simulink model "simu8"  (R2023b)
settings: Solver=VariableStepAuto  StartTime=0.0  StopTime=10.0  RelTol=1e-3
values from neighbouring files (symbols this model uses):
  b = 0.0012    [CFRO.m]    (also in parametros8.m)
  J = 0.001    [CFRO.m]    (also in parametros8.m)
  Ke = 0.01    [CFRO.m]    (also in parametros8.m)
  Kt = 0.01    [CFRO.m]    (also in parametros8.m)
  Lu = 0.023    [CFRO.m]    (also in parametros8.m)
  Ra = 2    [parametros8.m]

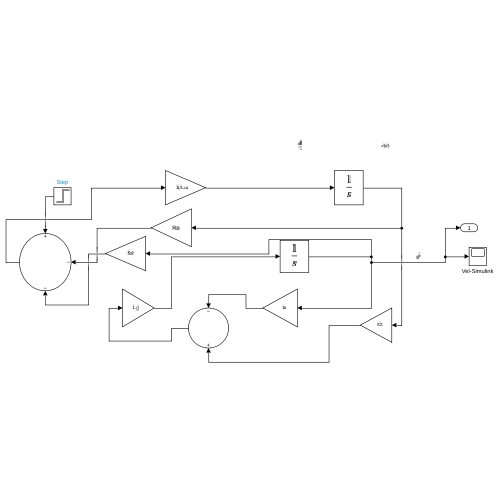
[thumbnail: Simulink's stored preview of the top-level diagram]
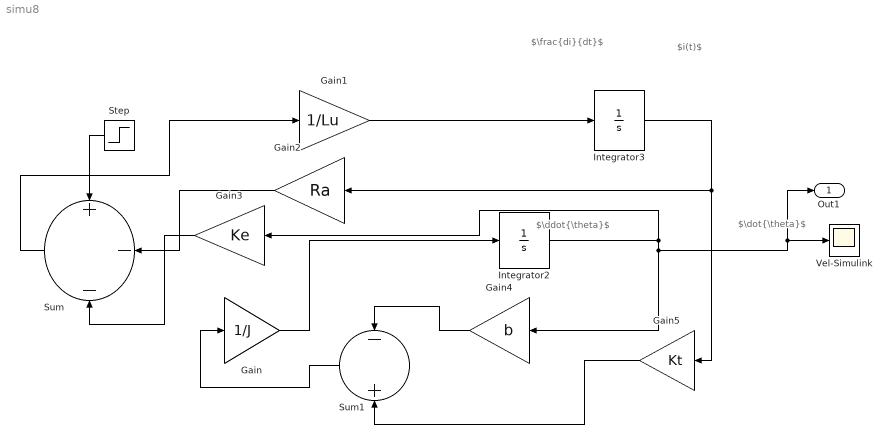
== system simu8 ==
  note: $\ddot{\theta}$
  note: $\frac{di}{dt}$
  note: $i(t)$
  note: $\dot{\theta}$
  Gain : Gain  Gain=1/J
  Gain1 : Gain  Gain=1/Lu
  Gain2 : Gain  Gain=Ra
  Gain3 : Gain  Gain=Ke
  Gain4 : Gain  Gain=b
  Gain5 : Gain  Gain=Kt
  Integrator2 : Integrator
  Integrator3 : Integrator
  Step : Step  Time=0  After=5  SampleTime=0
  Sum : Sum  Inputs=+--
  Sum1 : Sum  Inputs=-+
  Vel-Simulink : Scope
  Out1 : Outport
  wires:
  Step/1 -> Sum/1
  Sum1/1 -> Gain/1
  Integrator3/1 -> Gain5/1, Gain2/1
  Sum/1 -> Gain1/1
  Integrator2/1 -> Out1/1, Vel-Simulink/1, Gain4/1, Gain3/1
  Gain3/1 -> Sum/3
  Gain4/1 -> Sum1/1
  Gain5/1 -> Sum1/2
  Gain/1 -> Integrator2/1
  Gain1/1 -> Integrator3/1
  Gain2/1 -> Sum/2
